simulink model "pen_mpcpd"  (R2022b)
settings: Solver=VariableStepAuto  StartTime=0.0  StopTime=20  RelTol=1e-3  AbsTol=1e-3
settings Model: Creator=Abhijit  LastModifiedBy=abhij
settings SolverCC: AutoScaleAbsTol=off  AlgebraicLoopSolver=TrustRegion  MaxZcPerStep=1
settings DebuggingCC: UnconnectedInputMsg=warning  UnconnectedOutputMsg=warning  UnconnectedLineMsg=warning  SymbolicDimsDataTypeCodeGenerationDiagnostic=none  SFMachineParentedDataDiag=warning
settings ModelReferenceCC: EnableRefExpFcnMdlSchedulingChecks=on
settings SFSimCC: CustomCodeUndefinedFunction=UseInterfaceOnly
settings RTWCC: DLArmComputeVersion=19.05
settings SimscapeCC: SimscapeLogType=all  SimscapeLogSimulationStatistics=on  SimscapeLogDataHistory=10000

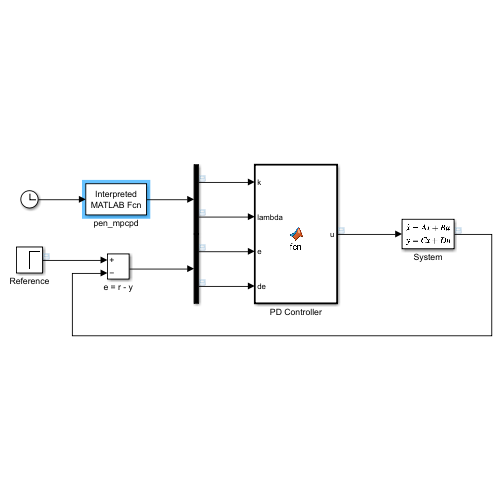
[thumbnail: Simulink's stored preview of the top-level diagram]
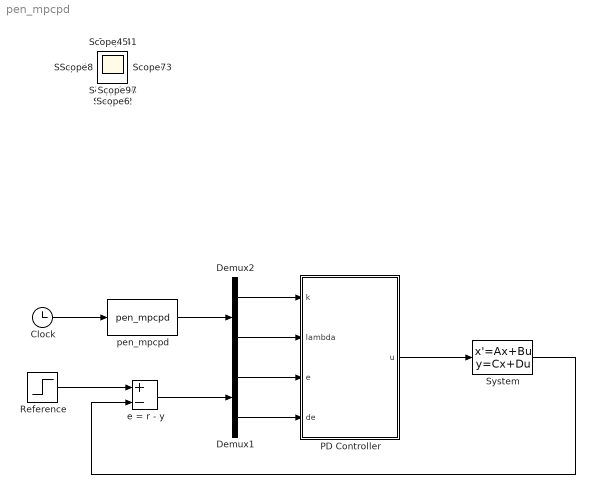
== system pen_mpcpd ==
  Clock : Clock
  Demux1 : Demux  Outputs=2
  Demux2 : Demux  Outputs=2
  PD Controller : MATLAB Function  TreatAsAtomicUnit=on
  Reference : Step  Before=[0; 0]  After=[0; pi]  SampleTime=0
  System : StateSpace  A=[0 -1; 1 0]  B=[1; 0]  C=[1 0; 0 1]  D=[0; 0]  InitialCondition=[0; 0]
  e = r - y : Sum  Inputs=+-
  pen_mpcpd : MATLABFcn  MATLABFcn=pen_mpcpd  OutputDimensions=2
  Scope{,1..45} (46 alike) : Scope
  wires:
  System/1 -> e = r - y/2
  Reference/1 -> e = r - y/1
  Demux1/1 -> PD Controller/3(e)
  Demux1/2 -> PD Controller/4(de)
  e = r - y/1 -> Demux1/1
  PD Controller/1(u) -> System/1
  Clock/1 -> pen_mpcpd/1
  Demux2/1 -> PD Controller/1(k)
  pen_mpcpd/1 -> Demux2/1
  Demux2/2 -> PD Controller/2(lambda)

== matlab function pen_mpcpd/PD Controller ==
  data: k input; lambda input; e input; u output; de input
function u = fcn(k, lambda, e, de)
    u = k*e + lambda*de;
end
